simulink model "MCCF_freq"  (Simulink 7.7)
settings: Solver=ode45  StartTime=0.0  StopTime=0.8  RelTol=1e-3
values from neighbouring files (symbols this model uses):
  ki = (wn^2)/Em    [PLL_Init_3approaches.m]    (also in PLL_Init_complete_without_recent_errata.m; approach_comp.m = (wn.^2)./Em; cardan_self_consistent.m; cardan_self_consistent_inbuiltsolve.m)
  kp = 2*del*wn/Em    [PLL_Init_3approaches.m]    (also in PLL_Init_complete_without_recent_errata.m; approach_comp.m = 2.*del.*wn/Em; cardan_self_consistent.m; cardan_self_consistent_inbuiltsolve.m)
  wc = w0/sqrt(2)    [MCCF_bode_mag_plots.m]    (also in PLL_Init_3approaches.m = 314.159265359; PLL_Init_complete_without_recent_errata.m = 314.159265359)
libraries: aerolibobsolete x1
settings Model: Creator=Sambhav  LastModifiedBy=Sambhav

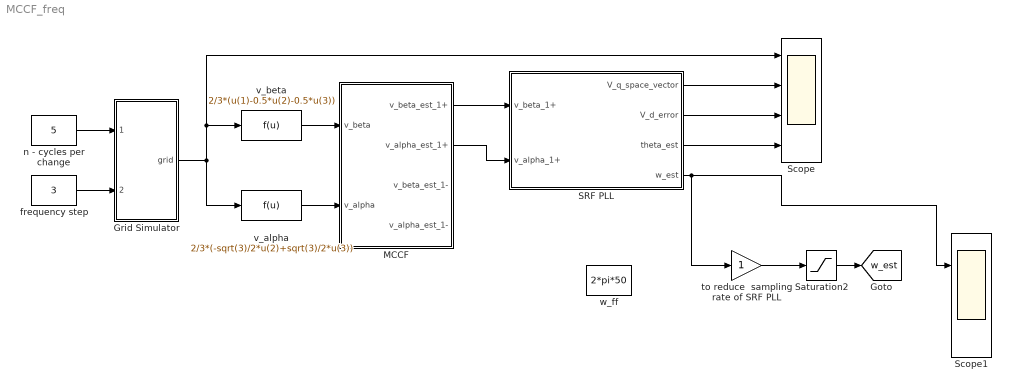
== system MCCF_freq ==
  Grid Simulator : Subsystem
  MCCF : Subsystem
  SRF PLL : Subsystem
  Saturation2 : Saturate  UpperLimit=2*pi*60  LowerLimit=2*pi*40
  Scope : Scope  NumInputPorts=4
      settings: TimeRange=0.8  YMin=-500~-4~294.8412698412699~-60  YMax=500~4~362.3015873015872~20  SampleInput=on  SampleTime=0.0001
  Scope1 : Scope  NumInputPorts=2
      settings: TimeRange=0.8  YMin=-500~-4  YMax=500~4  SampleInput=on  SampleTime=0.0001
  frequency step : Constant  Value=3
  n - cycles per change : Constant  Value=5
  to reduce  sampling rate of SRF PLL : Gain  SampleTime=0.01
  v_alpha : Fcn  Expr=2/3*(-sqrt(3)/2*u(2)+sqrt(3)/2*u(3))
  v_beta : Fcn  Expr=2/3*(u(1)-0.5*u(2)-0.5*u(3))
  w_ff : Constant  Value=2*pi*50
  tag scope: w_est=global
  wires:
  v_alpha/1 -> MCCF/2(v_alpha)
  v_beta/1 -> MCCF/1(v_beta)
  MCCF/1(v_beta_est_1+) -> SRF PLL/1(v_beta_1+)
  MCCF/2(v_alpha_est_1+) -> SRF PLL/2(v_alpha_1+)
  n - cycles per change/1 -> Grid Simulator/1(n cycles)
  frequency step/1 -> Grid Simulator/2(freq_step)
  Grid Simulator/1(grid) -> v_alpha/1, v_beta/1, Scope/1
  SRF PLL/1(V_q_space_vector) -> Scope/2
  SRF PLL/2(V_d_error) -> Scope/3
  SRF PLL/3(theta_est) -> Scope/4
  SRF PLL/4(w_est) -> Scope1/1, to reduce  sampling rate of SRF PLL/1
  to reduce  sampling rate of SRF PLL/1 -> Saturation2/1
  Saturation2/1 -> [w_est]

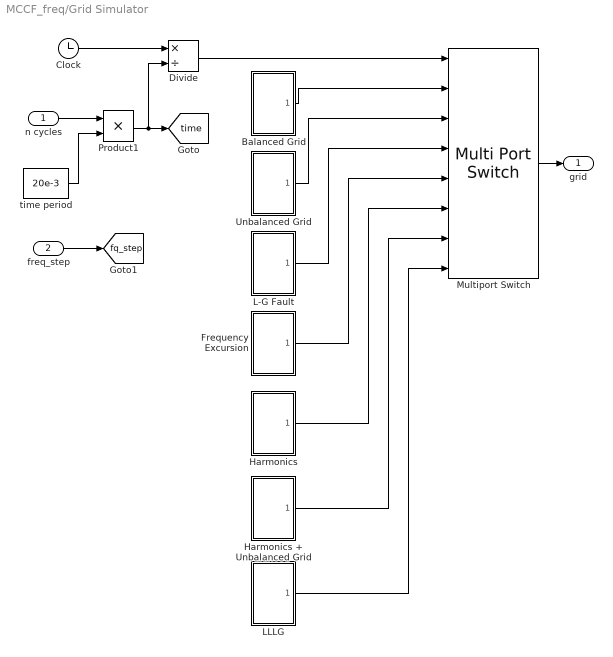
== system MCCF_freq/Grid Simulator ==
  n cycles : Inport
  freq_step : Inport  Port=2
  Balanced Grid : Subsystem
  Clock : Clock
  Divide : Product  Inputs=*/
  Frequency Excursion : Subsystem
  Harmonics : Subsystem
  Harmonics + Unbalanced Grid : Subsystem
  L-G Fault : Subsystem
  LLLG : Subsystem
  Multiport Switch : MultiPortSwitch  Inputs=7  DiagnosticForDefault=None  zeroidx=off
  Product1 : Product  RndMeth=Zero
  Unbalanced Grid : Subsystem
  time period : Constant  Value=20e-3
  grid : Outport
  tag scope: fq_step=global, time=global
  wires:
  Unbalanced Grid/1(v_grid) -> Multiport Switch/3
  Balanced Grid/1(v_grid) -> Multiport Switch/2
  L-G Fault/1(v_grid) -> Multiport Switch/4
  Frequency Excursion/1(v_grid) -> Multiport Switch/5
  Harmonics/1(v_grid) -> Multiport Switch/6
  Clock/1 -> Divide/1
  time period/1 -> Product1/2
  Product1/1 -> Divide/2, [time]
  Divide/1 -> Multiport Switch/1
  LLLG/1(v_grid) -> Multiport Switch/8
  Harmonics + Unbalanced Grid/1(v_grid) -> Multiport Switch/7
  n cycles/1 -> Product1/1
  Multiport Switch/1 -> grid/1
  freq_step/1 -> [fq_step]

== system MCCF_freq/MCCF ==
  v_beta : Inport
  v_alpha : Inport  Port=2
  Subsystem : Subsystem
  Sum : Sum  Inputs=|+-
  Sum1 : Sum  Inputs=|+-
  Sum2 : Sum  Inputs=+|+|+|+|+|+|+|+
  Sum6 : Sum  Inputs=+|+|+|+|+|+|+|+
  v_beta_est_1+ : Outport
  v_alpha_est_1+ : Outport  Port=2
  v_beta_est_1- : Outport  Port=3
  v_alpha_est_1- : Outport  Port=4
  wires:
  Sum2/1 -> Sum1/2
  Sum6/1 -> Sum/2
  Subsystem/16(v_alpha_est_11-) -> Sum2/8
  Subsystem/14(v_alpha_est_11+) -> Sum2/7
  Subsystem/12(v_alpha_est_7-) -> Sum2/6
  Subsystem/10(v_alpha_est_7+) -> Sum2/5
  Subsystem/8(v_alpha_est_5-) -> Sum2/4
  Subsystem/6(v_alpha_est_5+) -> Sum2/3
  Subsystem/4(v_alpha_est_1-) -> Sum2/2, v_alpha_est_1-/1
  Subsystem/2(v_alpha_est_1+) -> Sum2/1, v_alpha_est_1+/1
  Subsystem/15(v_beta_est_11-) -> Sum6/8
  Subsystem/13(v_beta_est_11+) -> Sum6/7
  Subsystem/11(v_beta_est_7-) -> Sum6/6
  Subsystem/9(v_beta_est_7+) -> Sum6/5
  Subsystem/7(v_beta_est_5-) -> Sum6/4
  Subsystem/5(v_beta_est_5+) -> Sum6/3
  Subsystem/3(v_beta_est_1-) -> Sum6/2, v_beta_est_1-/1
  Subsystem/1(v_beta_est_1+) -> Sum6/1, v_beta_est_1+/1
  Sum1/1 -> Subsystem/2(v_alpha_n)
  Sum/1 -> Subsystem/1(v_beta_n)
  v_beta/1 -> Sum/1
  v_alpha/1 -> Sum1/1

== system MCCF_freq/SRF PLL ==
  note: cos
  note: sin
  v_beta_1+ : Inport
  v_alpha_1+ : Inport  Port=2
  Integrator : Integrator
  Loop Filter : TransferFcn  Numerator=[kp ki]  Denominator=[1 0]
  Mux1 : Mux
  SinCos : aerolibobsolete/SinCos  SystemSampleTime=-1
  Sum : Sum  Inputs=|++
  Trigonometric Function : Trigonometry  Operator=atan2
  v_d : Fcn  Expr=u(1)*u(3)+u(2)*u(4)
  v_q : Fcn  Expr=u(1)*u(4)-u(2)*u(3)
  w_ff : Constant  Value=2*pi*50
  V_q_space_vector : Outport
  V_d_error : Outport  Port=2
  theta_est : Outport  Port=3
  w_est : Outport  Port=4
  wires:
  Loop Filter/1 -> Sum/1
  Sum/1 -> Integrator/1, w_est/1
  v_d/1 -> Loop Filter/1, V_d_error/1
  Integrator/1 -> SinCos/1
  Mux1/1 -> v_d/1, v_q/1
  SinCos/2 -> Mux1/4, Trigonometric Function/2
  SinCos/1 -> Mux1/3, Trigonometric Function/1
  v_beta_1+/1 -> Mux1/1
  v_alpha_1+/1 -> Mux1/2
  v_q/1 -> V_q_space_vector/1
  Trigonometric Function/1 -> theta_est/1
  w_ff/1 -> Sum/2

== system MCCF_freq/Grid Simulator/Balanced Grid ==
  Mux : Mux  Inputs=3
  v_a : Sin  Amplitude=230*sqrt(2)  Frequency=2*pi*50  Phase=pi/2  SampleTime=0
  v_b : Sin  Amplitude=230*sqrt(2)  Frequency=2*pi*50  Phase=pi/2-2*pi/3  SampleTime=0
  v_c : Sin  Amplitude=230*sqrt(2)  Frequency=2*pi*50  Phase=pi/2+2*pi/3  SampleTime=0
  v_grid : Outport
  wires:
  v_a/1 -> Mux/1
  v_b/1 -> Mux/2
  v_c/1 -> Mux/3
  Mux/1 -> v_grid/1

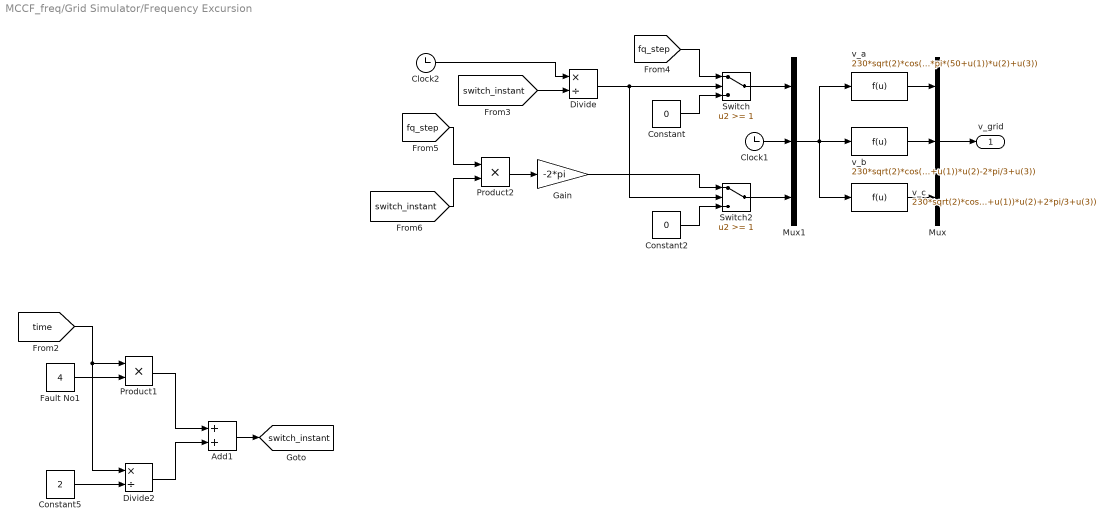
== system MCCF_freq/Grid Simulator/Frequency Excursion ==
  Add1 : Sum
  Clock1 : Clock
      settings: Decimation=10
  Clock2 : Clock
      settings: Decimation=10
  Constant : Constant  Value=0
  Constant2 : Constant  Value=0
  Constant5 : Constant  Value=2
  Divide : Product  Inputs=*/
  Divide2 : Product  Inputs=*/
  Fault No1 : Constant  Value=4
  Gain : Gain  Gain=-2*pi
  Mux : Mux  Inputs=3
  Mux1 : Mux  Inputs=3
  Product1 : Product  RndMeth=Zero
  Product2 : Product  RndMeth=Zero
  Switch : Switch  Threshold=1
  Switch2 : Switch  Threshold=1
  v_a : Fcn  Expr=230*sqrt(2)*cos(2*pi*(50+u(1))*u(2)+u(3))
  v_b : Fcn  Expr=230*sqrt(2)*cos(2*pi*(50+u(1))*u(2)-2*pi/3+u(3))
  v_c : Fcn  Expr=230*sqrt(2)*cos(2*pi*(50+u(1))*u(2)+2*pi/3+u(3))
  v_grid : Outport
  tag scope: switch_instant=global
  wires:
  [fq_step] -> Switch/1
  Constant/1 -> Switch/3
  Mux1/1 -> v_a/1, v_b/1, v_c/1
  v_a/1 -> Mux/1
  v_b/1 -> Mux/2
  v_c/1 -> Mux/3
  Constant2/1 -> Switch2/3
  Switch2/1 -> Mux1/3
  Gain/1 -> Switch2/1
  [time] -> Divide2/1, Product1/1
  Fault No1/1 -> Product1/2
  Product1/1 -> Add1/1
  Constant5/1 -> Divide2/2
  Divide2/1 -> Add1/2
  Mux/1 -> v_grid/1
  Switch/1 -> Mux1/1
  Clock2/1 -> Divide/1
  Add1/1 -> [switch_instant]
  [switch_instant] -> Divide/2
  Divide/1 -> Switch/2, Switch2/2
  [fq_step] -> Product2/1
  [switch_instant] -> Product2/2
  Product2/1 -> Gain/1
  Clock1/1 -> Mux1/2

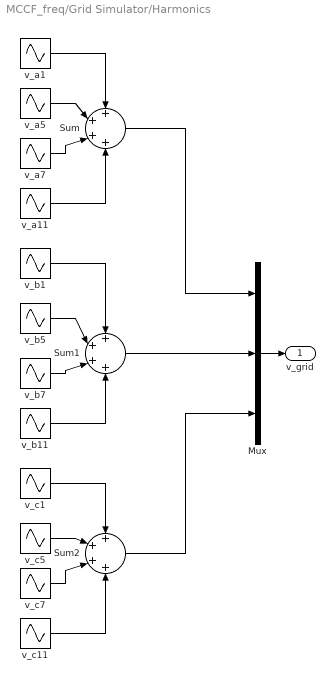
== system MCCF_freq/Grid Simulator/Harmonics ==
  Mux : Mux  Inputs=3
  Sum : Sum  Inputs=+|+|+|+
  Sum1 : Sum  Inputs=+|+|+|+
  Sum2 : Sum  Inputs=+|+|+|+
  v_a1 : Sin  Amplitude=230*sqrt(2)  Frequency=2*pi*50  Phase=pi/2  SampleTime=0
  v_a11 : Sin  Amplitude=230*sqrt(2)/11  Frequency=2*pi*50*11  Phase=pi/2  SampleTime=0
  v_a5 : Sin  Amplitude=230*sqrt(2)/5  Frequency=2*pi*50*5  Phase=pi/2  SampleTime=0
  v_a7 : Sin  Amplitude=230*sqrt(2)/7  Frequency=2*pi*50*7  Phase=pi/2  SampleTime=0
  v_b1 : Sin  Amplitude=230*sqrt(2)  Frequency=2*pi*50  Phase=pi/2-2*pi/3  SampleTime=0
  v_b11 : Sin  Amplitude=230*sqrt(2)/11  Frequency=2*pi*50*11  Phase=pi/2-2*pi/3  SampleTime=0
  v_b5 : Sin  Amplitude=230*sqrt(2)/5  Frequency=2*pi*50*5  Phase=pi/2-2*pi/3  SampleTime=0
  v_b7 : Sin  Amplitude=230*sqrt(2)/7  Frequency=2*pi*50*7  Phase=pi/2-2*pi/3  SampleTime=0
  v_c1 : Sin  Amplitude=230*sqrt(2)  Frequency=2*pi*50  Phase=pi/2+2*pi/3  SampleTime=0
  v_c11 : Sin  Amplitude=230*sqrt(2)/11  Frequency=2*pi*50*11  Phase=pi/2+2*pi/3  SampleTime=0
  v_c5 : Sin  Amplitude=230*sqrt(2)/5  Frequency=2*pi*50*5  Phase=pi/2+2*pi/3  SampleTime=0
  v_c7 : Sin  Amplitude=230*sqrt(2)/7  Frequency=2*pi*50*7  Phase=pi/2+2*pi/3  SampleTime=0
  v_grid : Outport
  wires:
  Mux/1 -> v_grid/1
  v_a1/1 -> Sum/1
  v_a5/1 -> Sum/2
  v_a7/1 -> Sum/3
  v_a11/1 -> Sum/4
  v_b1/1 -> Sum1/1
  v_b11/1 -> Sum1/4
  v_b5/1 -> Sum1/2
  v_b7/1 -> Sum1/3
  v_c1/1 -> Sum2/1
  v_c5/1 -> Sum2/2
  v_c7/1 -> Sum2/3
  v_c11/1 -> Sum2/4
  Sum/1 -> Mux/1
  Sum1/1 -> Mux/2
  Sum2/1 -> Mux/3

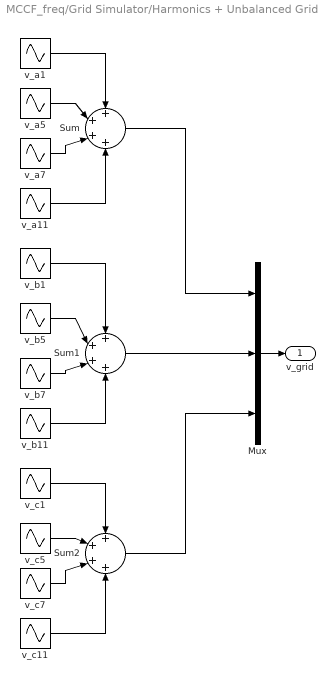
== system MCCF_freq/Grid Simulator/Harmonics + Unbalanced Grid ==
  Mux : Mux  Inputs=3
  Sum : Sum  Inputs=+|+|+|+
  Sum1 : Sum  Inputs=+|+|+|+
  Sum2 : Sum  Inputs=+|+|+|+
  v_a1 : Sin  Amplitude=230*sqrt(2)  Frequency=2*pi*50  Phase=pi/2  SampleTime=0
  v_a11 : Sin  Amplitude=230*sqrt(2)/11  Frequency=2*pi*50*11  Phase=pi/2  SampleTime=0
  v_a5 : Sin  Amplitude=230*sqrt(2)/5  Frequency=2*pi*50*5  Phase=pi/2  SampleTime=0
  v_a7 : Sin  Amplitude=230*sqrt(2)/7  Frequency=2*pi*50*7  Phase=pi/2  SampleTime=0
  v_b1 : Sin  Amplitude=200*sqrt(2)  Frequency=2*pi*50  Phase=pi/2-2*pi/3+pi/6  SampleTime=0
  v_b11 : Sin  Amplitude=220*sqrt(2)/11  Frequency=2*pi*50*11  Phase=pi/2-2*pi/3+pi/6  SampleTime=0
  v_b5 : Sin  Amplitude=200*sqrt(2)/5  Frequency=2*pi*50*5  Phase=pi/2-2*pi/3+pi/6  SampleTime=0
  v_b7 : Sin  Amplitude=200*sqrt(2)/7  Frequency=2*pi*50*7  Phase=pi/2-2*pi/3+pi/6  SampleTime=0
  v_c1 : Sin  Amplitude=210*sqrt(2)  Frequency=2*pi*50  Phase=pi/2+2*pi/3-pi/18  SampleTime=0
  v_c11 : Sin  Amplitude=210*sqrt(2)/11  Frequency=2*pi*50*11  Phase=pi/2+2*pi/3-pi/18  SampleTime=0
  v_c5 : Sin  Amplitude=210*sqrt(2)/5  Frequency=2*pi*50*5  Phase=pi/2+2*pi/3-pi/18  SampleTime=0
  v_c7 : Sin  Amplitude=210*sqrt(2)/7  Frequency=2*pi*50*7  Phase=pi/2+2*pi/3-pi/18  SampleTime=0
  v_grid : Outport
  wires:
  Sum2/1 -> Mux/3
  Sum1/1 -> Mux/2
  Sum/1 -> Mux/1
  v_c11/1 -> Sum2/4
  v_c7/1 -> Sum2/3
  v_c5/1 -> Sum2/2
  v_c1/1 -> Sum2/1
  v_b7/1 -> Sum1/3
  v_b5/1 -> Sum1/2
  v_b11/1 -> Sum1/4
  v_b1/1 -> Sum1/1
  v_a11/1 -> Sum/4
  v_a7/1 -> Sum/3
  v_a5/1 -> Sum/2
  v_a1/1 -> Sum/1
  Mux/1 -> v_grid/1

== system MCCF_freq/Grid Simulator/L-G Fault ==
  Mux : Mux  Inputs=3
  v_a : Sin  Amplitude=230*sqrt(2)  Frequency=2*pi*50  Phase=pi/2  SampleTime=0
  v_b : Sin  Amplitude=10  Frequency=2*pi*50  Phase=pi/2-2*pi/3  SampleTime=0
  v_c : Sin  Amplitude=230*sqrt(2)  Frequency=2*pi*50  Phase=pi/2+2*pi/3  SampleTime=0
  v_grid : Outport
  wires:
  Mux/1 -> v_grid/1
  v_c/1 -> Mux/3
  v_b/1 -> Mux/2
  v_a/1 -> Mux/1

== system MCCF_freq/Grid Simulator/LLLG ==
  Mux : Mux  Inputs=3
  v_a : Sin  Amplitude=0  Frequency=0  SampleTime=0
  v_b : Sin  Amplitude=0  Frequency=0  SampleTime=0
  v_c : Sin  Amplitude=0  Frequency=0  SampleTime=0
  v_grid : Outport
  wires:
  Mux/1 -> v_grid/1
  v_c/1 -> Mux/3
  v_b/1 -> Mux/2
  v_a/1 -> Mux/1

== system MCCF_freq/Grid Simulator/Unbalanced Grid ==
  Mux : Mux  Inputs=3
  v_a : Sin  Amplitude=230*sqrt(2)  Frequency=2*pi*50  Phase=pi/2  SampleTime=0
  v_b : Sin  Amplitude=200*sqrt(2)  Frequency=2*pi*50  Phase=pi/2-2*pi/3+pi/6  SampleTime=0
  v_c : Sin  Amplitude=210*sqrt(2)  Frequency=2*pi*50  Phase=pi/2+2*pi/3-pi/18  SampleTime=0
  v_grid : Outport
  wires:
  v_a/1 -> Mux/1
  v_b/1 -> Mux/2
  v_c/1 -> Mux/3
  Mux/1 -> v_grid/1

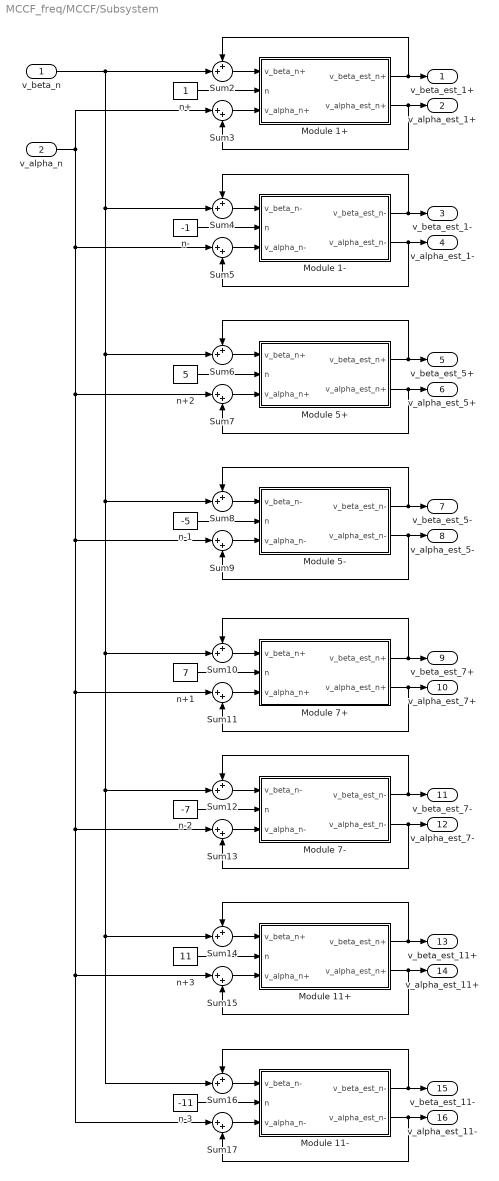
== system MCCF_freq/MCCF/Subsystem ==
  v_beta_n : Inport
  v_alpha_n : Inport  Port=2
  Module 1+ : Subsystem
  Module 1- : Subsystem
  Module 11+ : Subsystem
  Module 11- : Subsystem
  Module 5+ : Subsystem
  Module 5- : Subsystem
  Module 7+ : Subsystem
  Module 7- : Subsystem
  Sum{2,4,6,8,10,12,14,16} (8 alike) : Sum  Inputs=++|
  Sum{3,5,7,9,11,13,15,17} (8 alike) : Sum  Inputs=|++
  n+ : Constant
  n+1 : Constant  Value=7
  n+2 : Constant  Value=5
  n+3 : Constant  Value=11
  n- : Constant  Value=-1
  n-1 : Constant  Value=-5
  n-2 : Constant  Value=-7
  n-3 : Constant  Value=-11
  v_beta_est_1+ : Outport
  v_alpha_est_1+ : Outport  Port=2
  v_beta_est_1- : Outport  Port=3
  v_alpha_est_1- : Outport  Port=4
  v_beta_est_5+ : Outport  Port=5
  v_alpha_est_5+ : Outport  Port=6
  v_beta_est_5- : Outport  Port=7
  v_alpha_est_5- : Outport  Port=8
  v_beta_est_7+ : Outport  Port=9
  v_alpha_est_7+ : Outport  Port=10
  v_beta_est_7- : Outport  Port=11
  v_alpha_est_7- : Outport  Port=12
  v_beta_est_11+ : Outport  Port=13
  v_alpha_est_11+ : Outport  Port=14
  v_beta_est_11- : Outport  Port=15
  v_alpha_est_11- : Outport  Port=16
  wires:
  n+/1 -> Module 1+/2(n)
  Sum2/1 -> Module 1+/1(v_beta_n+)
  Sum3/1 -> Module 1+/3(v_alpha_n+)
  Module 1+/1(v_beta_est_n+) -> Sum2/1, v_beta_est_1+/1
  Module 1+/2(v_alpha_est_n+) -> Sum3/2, v_alpha_est_1+/1
  n-/1 -> Module 1-/2(n)
  Sum4/1 -> Module 1-/1(v_beta_n-)
  Sum5/1 -> Module 1-/3(v_alpha_n-)
  Module 1-/1(v_beta_est_n-) -> Sum4/1, v_beta_est_1-/1
  Module 1-/2(v_alpha_est_n-) -> Sum5/2, v_alpha_est_1-/1
  n+2/1 -> Module 5+/2(n)
  Sum6/1 -> Module 5+/1(v_beta_n+)
  Sum7/1 -> Module 5+/3(v_alpha_n+)
  Module 5+/1(v_beta_est_n+) -> Sum6/1, v_beta_est_5+/1
  Module 5+/2(v_alpha_est_n+) -> Sum7/2, v_alpha_est_5+/1
  n-1/1 -> Module 5-/2(n)
  Sum8/1 -> Module 5-/1(v_beta_n-)
  Sum9/1 -> Module 5-/3(v_alpha_n-)
  Module 5-/1(v_beta_est_n-) -> Sum8/1, v_beta_est_5-/1
  Module 5-/2(v_alpha_est_n-) -> Sum9/2, v_alpha_est_5-/1
  n+1/1 -> Module 7+/2(n)
  Sum10/1 -> Module 7+/1(v_beta_n+)
  Sum11/1 -> Module 7+/3(v_alpha_n+)
  Module 7+/1(v_beta_est_n+) -> Sum10/1, v_beta_est_7+/1
  Module 7+/2(v_alpha_est_n+) -> Sum11/2, v_alpha_est_7+/1
  n-2/1 -> Module 7-/2(n)
  Sum12/1 -> Module 7-/1(v_beta_n-)
  Sum13/1 -> Module 7-/3(v_alpha_n-)
  Module 7-/1(v_beta_est_n-) -> Sum12/1, v_beta_est_7-/1
  Module 7-/2(v_alpha_est_n-) -> Sum13/2, v_alpha_est_7-/1
  n+3/1 -> Module 11+/2(n)
  Sum14/1 -> Module 11+/1(v_beta_n+)
  Sum15/1 -> Module 11+/3(v_alpha_n+)
  Module 11+/1(v_beta_est_n+) -> Sum14/1, v_beta_est_11+/1
  Module 11+/2(v_alpha_est_n+) -> Sum15/2, v_alpha_est_11+/1
  n-3/1 -> Module 11-/2(n)
  Sum16/1 -> Module 11-/1(v_beta_n-)
  Sum17/1 -> Module 11-/3(v_alpha_n-)
  Module 11-/1(v_beta_est_n-) -> Sum16/1, v_beta_est_11-/1
  Module 11-/2(v_alpha_est_n-) -> Sum17/2, v_alpha_est_11-/1
  v_beta_n/1 -> Sum16/2, Sum14/2, Sum12/2, Sum10/2, Sum8/2, Sum6/2, Sum4/2, Sum2/2
  v_alpha_n/1 -> Sum17/1, Sum15/1, Sum13/1, Sum11/1, Sum9/1, Sum7/1, Sum5/1, Sum3/1

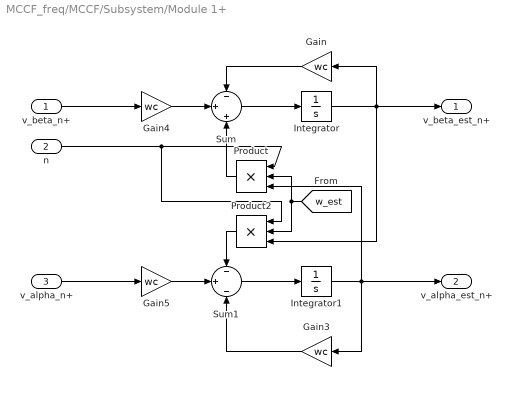
== system MCCF_freq/MCCF/Subsystem/Module 1+ ==
  v_beta_n+ : Inport
  n : Inport  Port=2
  v_alpha_n+ : Inport  Port=3
  Gain{,3..5} (4 alike) : Gain  Gain=wc
  Integrator : Integrator
  Integrator1 : Integrator
  Product : Product  Inputs=3  RndMeth=Zero
  Product2 : Product  Inputs=3  RndMeth=Zero
  Sum : Sum  Inputs=-|+|+
  Sum1 : Sum  Inputs=-|+|-
  v_beta_est_n+ : Outport
  v_alpha_est_n+ : Outport  Port=2
  wires:
  Gain3/1 -> Sum1/3
  Gain/1 -> Sum/1
  Gain4/1 -> Sum/2
  Gain5/1 -> Sum1/2
  Sum1/1 -> Integrator1/1
  Sum/1 -> Integrator/1
  Integrator1/1 -> Gain3/1, v_alpha_est_n+/1, Product/3
  Integrator/1 -> Gain/1, v_beta_est_n+/1, Product2/3
  Product/1 -> Sum/3
  Product2/1 -> Sum1/1
  n/1 -> Product/1, Product2/1
  v_beta_n+/1 -> Gain4/1
  v_alpha_n+/1 -> Gain5/1
  [w_est] -> Product/2, Product2/2

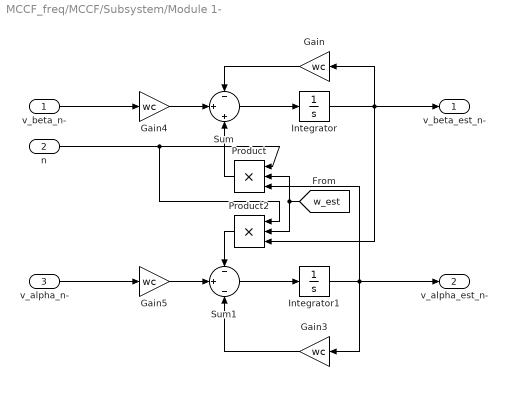
== system MCCF_freq/MCCF/Subsystem/Module 1- ==
  v_beta_n- : Inport
  n : Inport  Port=2
  v_alpha_n- : Inport  Port=3
  Gain{,3..5} (4 alike) : Gain  Gain=wc
  Integrator : Integrator
  Integrator1 : Integrator
  Product : Product  Inputs=3  RndMeth=Zero
  Product2 : Product  Inputs=3  RndMeth=Zero
  Sum : Sum  Inputs=-|+|+
  Sum1 : Sum  Inputs=-|+|-
  v_beta_est_n- : Outport
  v_alpha_est_n- : Outport  Port=2
  wires:
  [w_est] -> Product2/2, Product/2
  v_alpha_n-/1 -> Gain5/1
  v_beta_n-/1 -> Gain4/1
  n/1 -> Product2/1, Product/1
  Product2/1 -> Sum1/1
  Product/1 -> Sum/3
  Integrator/1 -> Product2/3, v_beta_est_n-/1, Gain/1
  Integrator1/1 -> Product/3, v_alpha_est_n-/1, Gain3/1
  Sum/1 -> Integrator/1
  Sum1/1 -> Integrator1/1
  Gain5/1 -> Sum1/2
  Gain4/1 -> Sum/2
  Gain/1 -> Sum/1
  Gain3/1 -> Sum1/3

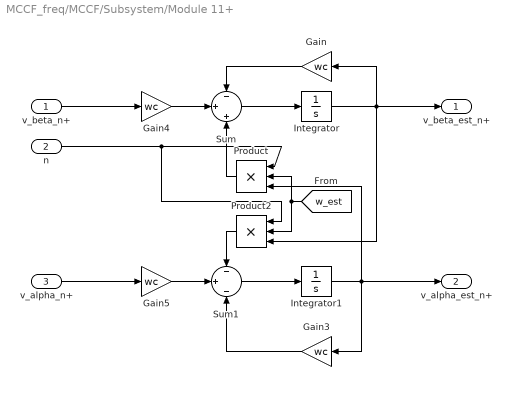
== system MCCF_freq/MCCF/Subsystem/Module 11+ ==
  v_beta_n+ : Inport
  n : Inport  Port=2
  v_alpha_n+ : Inport  Port=3
  Gain{,3..5} (4 alike) : Gain  Gain=wc
  Integrator : Integrator
  Integrator1 : Integrator
  Product : Product  Inputs=3  RndMeth=Zero
  Product2 : Product  Inputs=3  RndMeth=Zero
  Sum : Sum  Inputs=-|+|+
  Sum1 : Sum  Inputs=-|+|-
  v_beta_est_n+ : Outport
  v_alpha_est_n+ : Outport  Port=2
  wires:
  [w_est] -> Product2/2, Product/2
  v_alpha_n+/1 -> Gain5/1
  v_beta_n+/1 -> Gain4/1
  n/1 -> Product2/1, Product/1
  Product2/1 -> Sum1/1
  Product/1 -> Sum/3
  Integrator/1 -> Product2/3, v_beta_est_n+/1, Gain/1
  Integrator1/1 -> Product/3, v_alpha_est_n+/1, Gain3/1
  Sum/1 -> Integrator/1
  Sum1/1 -> Integrator1/1
  Gain5/1 -> Sum1/2
  Gain4/1 -> Sum/2
  Gain/1 -> Sum/1
  Gain3/1 -> Sum1/3

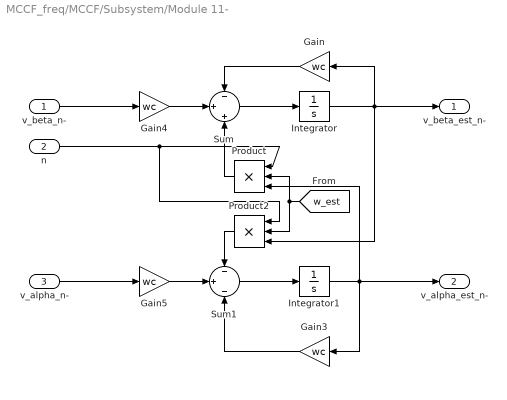
== system MCCF_freq/MCCF/Subsystem/Module 11- ==
  v_beta_n- : Inport
  n : Inport  Port=2
  v_alpha_n- : Inport  Port=3
  Gain{,3..5} (4 alike) : Gain  Gain=wc
  Integrator : Integrator
  Integrator1 : Integrator
  Product : Product  Inputs=3  RndMeth=Zero
  Product2 : Product  Inputs=3  RndMeth=Zero
  Sum : Sum  Inputs=-|+|+
  Sum1 : Sum  Inputs=-|+|-
  v_beta_est_n- : Outport
  v_alpha_est_n- : Outport  Port=2
  wires:
  Gain3/1 -> Sum1/3
  Gain/1 -> Sum/1
  Gain4/1 -> Sum/2
  Gain5/1 -> Sum1/2
  Sum1/1 -> Integrator1/1
  Sum/1 -> Integrator/1
  Integrator1/1 -> Gain3/1, v_alpha_est_n-/1, Product/3
  Integrator/1 -> Gain/1, v_beta_est_n-/1, Product2/3
  Product/1 -> Sum/3
  Product2/1 -> Sum1/1
  n/1 -> Product/1, Product2/1
  v_beta_n-/1 -> Gain4/1
  v_alpha_n-/1 -> Gain5/1
  [w_est] -> Product/2, Product2/2

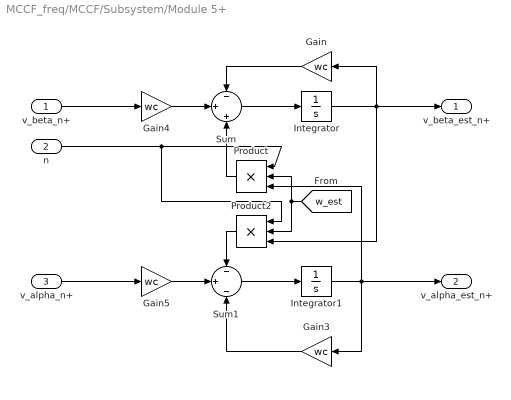
== system MCCF_freq/MCCF/Subsystem/Module 5+ ==
  v_beta_n+ : Inport
  n : Inport  Port=2
  v_alpha_n+ : Inport  Port=3
  Gain{,3..5} (4 alike) : Gain  Gain=wc
  Integrator : Integrator
  Integrator1 : Integrator
  Product : Product  Inputs=3  RndMeth=Zero
  Product2 : Product  Inputs=3  RndMeth=Zero
  Sum : Sum  Inputs=-|+|+
  Sum1 : Sum  Inputs=-|+|-
  v_beta_est_n+ : Outport
  v_alpha_est_n+ : Outport  Port=2
  wires:
  [w_est] -> Product2/2, Product/2
  v_alpha_n+/1 -> Gain5/1
  v_beta_n+/1 -> Gain4/1
  n/1 -> Product2/1, Product/1
  Product2/1 -> Sum1/1
  Product/1 -> Sum/3
  Integrator/1 -> Product2/3, v_beta_est_n+/1, Gain/1
  Integrator1/1 -> Product/3, v_alpha_est_n+/1, Gain3/1
  Sum/1 -> Integrator/1
  Sum1/1 -> Integrator1/1
  Gain5/1 -> Sum1/2
  Gain4/1 -> Sum/2
  Gain/1 -> Sum/1
  Gain3/1 -> Sum1/3

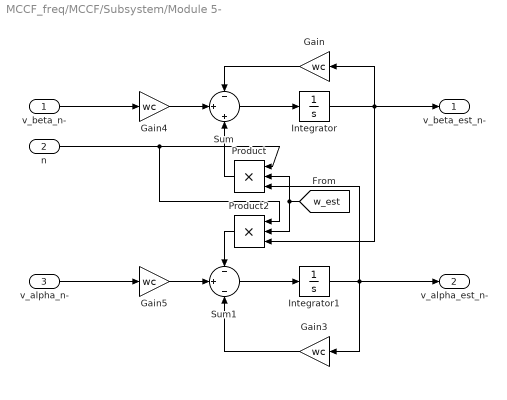
== system MCCF_freq/MCCF/Subsystem/Module 5- ==
  v_beta_n- : Inport
  n : Inport  Port=2
  v_alpha_n- : Inport  Port=3
  Gain{,3..5} (4 alike) : Gain  Gain=wc
  Integrator : Integrator
  Integrator1 : Integrator
  Product : Product  Inputs=3  RndMeth=Zero
  Product2 : Product  Inputs=3  RndMeth=Zero
  Sum : Sum  Inputs=-|+|+
  Sum1 : Sum  Inputs=-|+|-
  v_beta_est_n- : Outport
  v_alpha_est_n- : Outport  Port=2
  wires:
  Gain3/1 -> Sum1/3
  Gain/1 -> Sum/1
  Gain4/1 -> Sum/2
  Gain5/1 -> Sum1/2
  Sum1/1 -> Integrator1/1
  Sum/1 -> Integrator/1
  Integrator1/1 -> Gain3/1, v_alpha_est_n-/1, Product/3
  Integrator/1 -> Gain/1, v_beta_est_n-/1, Product2/3
  Product/1 -> Sum/3
  Product2/1 -> Sum1/1
  n/1 -> Product/1, Product2/1
  v_beta_n-/1 -> Gain4/1
  v_alpha_n-/1 -> Gain5/1
  [w_est] -> Product/2, Product2/2

== system MCCF_freq/MCCF/Subsystem/Module 7+ ==
  v_beta_n+ : Inport
  n : Inport  Port=2
  v_alpha_n+ : Inport  Port=3
  Gain{,3..5} (4 alike) : Gain  Gain=wc
  Integrator : Integrator
  Integrator1 : Integrator
  Product : Product  Inputs=3  RndMeth=Zero
  Product2 : Product  Inputs=3  RndMeth=Zero
  Sum : Sum  Inputs=-|+|+
  Sum1 : Sum  Inputs=-|+|-
  v_beta_est_n+ : Outport
  v_alpha_est_n+ : Outport  Port=2
  wires:
  Gain3/1 -> Sum1/3
  Gain/1 -> Sum/1
  Gain4/1 -> Sum/2
  Gain5/1 -> Sum1/2
  Sum1/1 -> Integrator1/1
  Sum/1 -> Integrator/1
  Integrator1/1 -> Gain3/1, v_alpha_est_n+/1, Product/3
  Integrator/1 -> Gain/1, v_beta_est_n+/1, Product2/3
  Product/1 -> Sum/3
  Product2/1 -> Sum1/1
  n/1 -> Product/1, Product2/1
  v_beta_n+/1 -> Gain4/1
  v_alpha_n+/1 -> Gain5/1
  [w_est] -> Product/2, Product2/2

== system MCCF_freq/MCCF/Subsystem/Module 7- ==
  v_beta_n- : Inport
  n : Inport  Port=2
  v_alpha_n- : Inport  Port=3
  Gain{,3..5} (4 alike) : Gain  Gain=wc
  Integrator : Integrator
  Integrator1 : Integrator
  Product : Product  Inputs=3  RndMeth=Zero
  Product2 : Product  Inputs=3  RndMeth=Zero
  Sum : Sum  Inputs=-|+|+
  Sum1 : Sum  Inputs=-|+|-
  v_beta_est_n- : Outport
  v_alpha_est_n- : Outport  Port=2
  wires:
  [w_est] -> Product2/2, Product/2
  v_alpha_n-/1 -> Gain5/1
  v_beta_n-/1 -> Gain4/1
  n/1 -> Product2/1, Product/1
  Product2/1 -> Sum1/1
  Product/1 -> Sum/3
  Integrator/1 -> Product2/3, v_beta_est_n-/1, Gain/1
  Integrator1/1 -> Product/3, v_alpha_est_n-/1, Gain3/1
  Sum/1 -> Integrator/1
  Sum1/1 -> Integrator1/1
  Gain5/1 -> Sum1/2
  Gain4/1 -> Sum/2
  Gain/1 -> Sum/1
  Gain3/1 -> Sum1/3
